simulink model "pwm_sc_motor"  (R2018b)
settings: Solver=ode15s  StartTime=0.0  StopTime=10  RelTol=1e-3  AbsTol=1e-3  EnableMultiTasking=on
values from neighbouring files (symbols this model uses):
  DC_Motor_J = 0.05    [dc_motor_script.m]    (also in values_01.mat = 0.0586707103924; values_02.mat = 0.038999801486)
libraries: fl_lib x6, nesl_utility x4, elec_lib x3
CloseFcn:
  | try,close(h1_elec_motor_dc_pwm),end
  | clear h1_elec_motor_dc_pwm
  | 
  | clear simlog_elec_motor_dc_pwm
  | clear logsout_elec_motor_dc_pwm
  | clear RPM RPM1 tout
Description:
  | PWM-Controlled DC Motor
  | 
  | Copyright 2008-2018 The MathWorks, Inc.
settings Model: Creator=MathWorks  LastModifiedBy=EDU_UGEX_7219
settings SolverCC: AutoScaleAbsTol=off
settings DataIOCC: LimitDataPoints=on  MaxDataPoints=10000  SaveFormat=Array  SignalLoggingSaveFormat=ModelDataLogs  SignalLoggingName=logsout_elec_motor_dc_pwm
settings OptimizationCC: ExpressionDepthLimit=2147483647  InitFltsAndDblsToZero=on  LifeSpan=inf
settings DebuggingCC: UnderspecifiedInitializationDetection=Classic  MergeDetectMultiDrivingBlocksExec=none  FcnCallInpInsideContextMsg=warning  StateNameClashWarn=warning  LibraryContextMissingDiagnostic=none  SFUnexpectedBacktrackingDiag=warning  SFNoUnconditionalDefaultTransitionDiag=warning  SFExecutionAtInitializationDiag=none
settings HardwareCC: ProdBitPerPointer=32  ProdBitPerSizeT=32  ProdBitPerPtrDiffT=32  ProdLargestAtomicFloat=None  ProdIntDivRoundTo=Undefined  ProdEndianess=Unspecified  ProdWordSize=32  ProdHWDeviceType=32-bit Generic
settings ModelReferenceCC: PropagateSignalLabelsOutOfModel=off
settings SFSimCC: SimUseLocalCustomCode=off
settings RTWCC: RTWUseLocalCustomCode=off
settings CodeAppCC: StateflowObjectComments=on
settings GRTTargetCC: TargetLangStandard=C89/C90 (ANSI)  GeneratePreprocessorConditionals=Disable all  CombineOutputUpdateFcns=off  GRTInterface=on
settings ConfigComp: CovMetricSettings=dw  CovHtmlReporting=on  CovSaveCumulativeToWorkspaceVar=on  CovSaveSingleToWorkspaceVar=on  CovExternalEMLEnable=off  CovSFcnEnable=off
settings SimscapeCC: SimscapeLogType=all  SimscapeLogSimulationStatistics=on  SimscapeLogName=simlog_elec_motor_dc_pwm  SimscapeLogDataHistory=10000

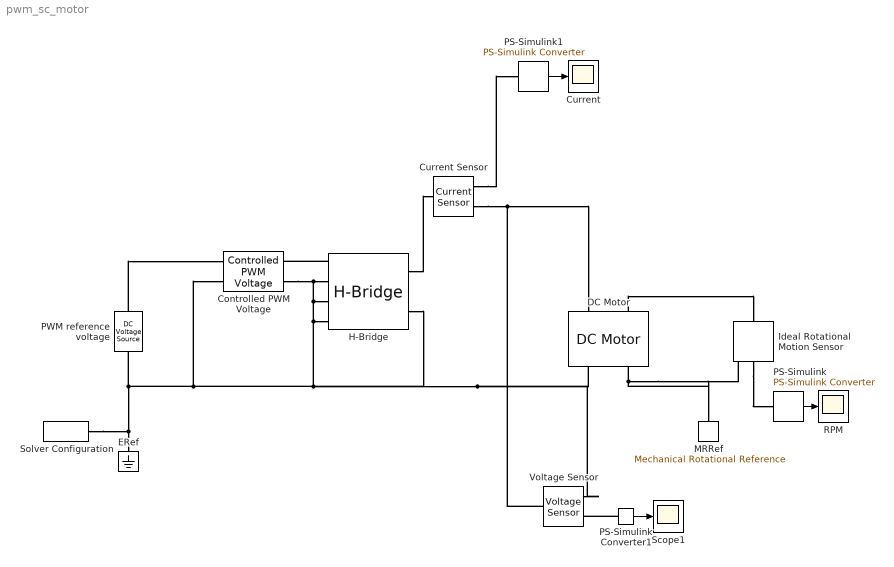
== system pwm_sc_motor ==
  Controlled PWM Voltage : elec_lib/Actuators & Drivers/Drivers/Controlled PWM Voltage  F=4000 Hz  TD=0 s  pulse_width_offset=0 s  pulse_min=0 s  Vmin=0 V  Vmax=5 V  Vm=5 V  pwm_or_av=2  event_type=1  sample_time=1e-6 s  u_min=0  u_max=1
      settings: SourceProductName=Simscape Electronics  SourceProductBaseCode=SN
  Current : Scope
  Current Sensor : fl_lib/Electrical/Electrical Sensors/Current Sensor
      settings: SourceProductName=Foundation Library
  DC Motor : elec_lib/Actuators & Drivers/Rotational Actuators/DC Motor  parameterization=1  Ra=DC_Motor_R Ohm  La=DC_Motor_L H  emf_or_torque=1  Kv=DC_Motor_K V/(rad/s)  Ki=6.876e-04 N*m/A  T_stall=0.1 N*m  w_max=4000 rpm  w_rated=2500 rpm  P_rated=10 W  V_rated=12 V  J=DC_Motor_J kg*m^2  lam_param=1  lam=DC_Motor_B N*m/(rad/s)  i_noload=0 A  V_i_noload=1.5 V  speed0=0 rpm  alpha=0.00393 1/K  Tmeas=25 degC  thermal_mass=100 J/K  initial_temperature=25 degC
  ERef : fl_lib/Electrical/Electrical Elements/Electrical Reference
      settings: SourceProductName=Foundation Library
  H-Bridge : elec_lib/Actuators & Drivers/Drivers/H-Bridge  Venable=2.5 V  Vmax=5 V  Vreverse=2.5 V  Vbrake=2.5 V  Vm=1 V  pwm_or_av=2  discontinuous=0  freewheeling_mode=1  freewheeling_mode_disc=1  Ron=0.1 Ohm  Don=0.1 Ohm  Rload=3.38+0.1 Ohm  Lload=1e-5 H  F=4 kHz  thermal_mass=100 J/K  initial_temperature=298.15 K  Ron2=0.1 Ohm  Don2=0.05 Ohm  Tmeas=298.15 K  Tmeas2=398.15 K
      settings: SourceProductName=Simscape Electronics  SourceProductBaseCode=SN
  Ideal Rotational Motion Sensor : fl_lib/Mechanical/Mechanical Sensors/Ideal Rotational Motion Sensor  offset=0 deg
      settings: SourceProductName=Foundation Library
  MRRef : fl_lib/Mechanical/Rotational Elements/Mechanical Rotational Reference
      settings: SourceProductName=Foundation Library
  PS-Simulink : nesl_utility/PS-Simulink Converter  PhysicalDomain=network_engine_domain  SubClassName=ps_output  LeftPortType=input  RightPortType=output  PseudoPeriodic=off  Frequencies=[]  Unit=rpm  AffineConversion=off
  PS-Simulink Converter1 : nesl_utility/PS-Simulink Converter  PhysicalDomain=network_engine_domain  SubClassName=ps_output  LeftPortType=input  RightPortType=output  PseudoPeriodic=off  Frequencies=[]  Unit=V  AffineConversion=off
  PS-Simulink1 : nesl_utility/PS-Simulink Converter  PhysicalDomain=network_engine_domain  SubClassName=ps_output  LeftPortType=input  RightPortType=output  PseudoPeriodic=off  Frequencies=[]  Unit=A  AffineConversion=off
  PWM reference voltage : fl_lib/Electrical/Electrical Sources/DC Voltage Source  v0=5 V
      settings: SourceProductName=Foundation Library
  RPM : Scope
  Scope1 : Scope
  Solver Configuration : nesl_utility/Solver Configuration  PhysicalDomain=network_engine_domain  SubClassName=solver  LeftPortType=input  RightPortType=generic  Tones=[]  Harmonics=[]  SimulateNoise=off  Profile=off  UseLocalSampling=off  EnableSwitchedLinearOptims=on  FrequencyDomain=off  UseCCode=off  RelTol=0.001  AbsTol=1e-06  MinStep=1e-09  ToWorkspace=off  RevertToSquareIcSolve=off  NumHomotopyIterations=100  PhasorMode=off  PhasorModeNumHarmonics=1  DoDC=off  ResidualTolerance=1e-9  UseLocalSolver=off  LocalSolverChoice=NE_BACKWARD_EULER_ADVANCER  LocalSolverSampleTime=.001  DoFixedCost=off  MaxNonlinIter=3  MaxModeIter=2  LinearAlgebra=auto  EquationFormulation=NE_TIME_EF  DelaysMemoryBudget=1024  AutomaticFiltering=on  FilteringTimeConstant=0.001  PartitionStorageMethod=AS_NEEDED  PartitionMemoryBudget=1024
  Voltage Sensor : fl_lib/Electrical/Electrical Sensors/Voltage Sensor
  wires:
  PS-Simulink/1 -> RPM/1
  PS-Simulink1/1 -> Current/1
  PS-Simulink Converter1/1 -> Scope1/1
  connections:
  DC Motor/LConn2 -- Ideal Rotational Motion Sensor/LConn1
  H-Bridge/LConn1 -- Controlled PWM Voltage/RConn1
  DC Motor/RConn2 -- MRRef/LConn1 -- Ideal Rotational Motion Sensor/RConn1
  Ideal Rotational Motion Sensor/RConn2 -- PS-Simulink/LConn1
  PWM reference voltage/LConn1 -- Controlled PWM Voltage/LConn1
  H-Bridge/RConn1 -- Current Sensor/LConn1
  Current Sensor/RConn2 -- Voltage Sensor/LConn1 -- DC Motor/LConn1
  Current Sensor/RConn1 -- PS-Simulink1/LConn1
  Voltage Sensor/RConn2 -- DC Motor/RConn1 -- H-Bridge/RConn2 -- ERef/LConn1 -- Solver Configuration/RConn1 -- PWM reference voltage/RConn1 -- Controlled PWM Voltage/LConn2 -- H-Bridge/LConn2 -- Controlled PWM Voltage/RConn2 -- H-Bridge/LConn3 -- H-Bridge/LConn4
  PS-Simulink Converter1/LConn1 -- Voltage Sensor/RConn1
